simulink model "quad_sim"  (R2016a)
settings: Solver=FixedStepAuto  StartTime=0.0  StopTime=T_sim  FixedStep=dt_sim  RelTol=1e-3
InitFcn:
  | %cd /home/adrianomcr/ROS_projects/vecfield_ws/src/vecfield_lib/simulink/quadrotor
  | MAV_constants
StopFcn:
  | animation
values from neighbouring files (symbols this model uses):
  curva = 9    [MAV_constants.m]
  Delta_omega = 0.5    [MAV_constants.m]
  Delta_tau = 1.0    (= 1)    [MAV_constants.m]
  drag_coef = 0.05    [MAV_constants.m]
  g = 9.81    [MAV_constants.m]
  Kf = 1    [MAV_constants.m]
  Kr = 5    [MAV_constants.m]
  Kv = 2    [MAV_constants.m]
  m = 0.5    [MAV_constants.m]
  Rot_0 = eul2rotm(fliplr([pi/4 pi/2 pi]))    [MAV_constants.m]
  vr = 4    [MAV_constants.m]
  xyz_0 = [-2 -2 -2] + 0.001    [MAV_constants.m]
  xyz_d_0 = [0 1 0] + 0.001    [MAV_constants.m]
settings Model: Creator=root  LastModifiedBy=adrianomcr

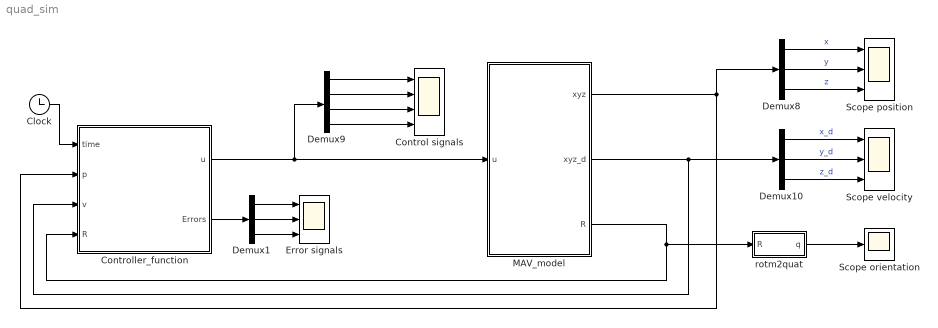
== system quad_sim ==
  Clock : Clock
  Control signals : Scope  NumInputPorts=4
  Controller_function : MATLAB Function  TreatAsAtomicUnit=on
  Demux1 : Demux  Outputs=3
  Demux10 : Demux  Outputs=3
  Demux8 : Demux  Outputs=3
  Demux9 : Demux
  Error signals : Scope  NumInputPorts=3
  MAV_model : Subsystem
  Scope orientation : Scope
  Scope position : Scope  NumInputPorts=3
  Scope velocity : Scope  NumInputPorts=3
  rotm2quat : MATLAB Function  TreatAsAtomicUnit=on
  wires:
  Demux8/1 -> Scope position/1  "x"
  Demux8/2 -> Scope position/2  "y"
  Demux8/3 -> Scope position/3  "z"
  Demux10/1 -> Scope velocity/1  "x_d"
  Demux10/2 -> Scope velocity/2  "y_d"
  Demux10/3 -> Scope velocity/3  "z_d"
  MAV_model/1(xyz) -> Demux8/1, Controller_function/2(p)
  MAV_model/2(xyz_d) -> Controller_function/3(v), Demux10/1
  MAV_model/3(R) -> Controller_function/4(R), rotm2quat/1(R)
  Controller_function/1(u) -> Demux9/1, MAV_model/1(u)
  Demux9/1 -> Control signals/1
  Demux9/2 -> Control signals/2
  Demux9/3 -> Control signals/3
  Demux9/4 -> Control signals/4
  Controller_function/2(Errors) -> Demux1/1
  Demux1/1 -> Error signals/1
  Demux1/2 -> Error signals/2
  Demux1/3 -> Error signals/3
  Clock/1 -> Controller_function/1(time)
  rotm2quat/1(q) -> Scope orientation/1

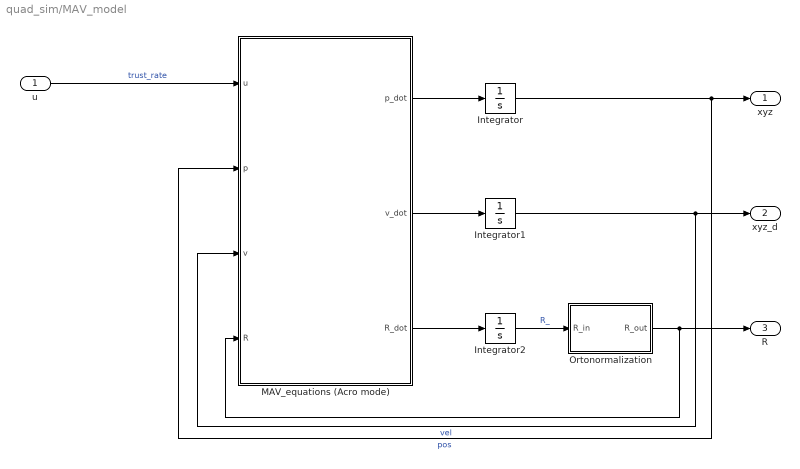
== system quad_sim/MAV_model ==
  u : Inport
  Integrator : Integrator  InitialCondition=xyz_0
  Integrator1 : Integrator  InitialCondition=xyz_d_0
  Integrator2 : Integrator  InitialCondition=Rot_0
  MAV_equations (Acro mode) : MATLAB Function  TreatAsAtomicUnit=on
  Ortonormalization : MATLAB Function  TreatAsAtomicUnit=on
  xyz : Outport
  xyz_d : Outport  Port=2
  R : Outport  Port=3
  wires:
  MAV_equations (Acro mode)/1(p_dot) -> Integrator/1
  MAV_equations (Acro mode)/2(v_dot) -> Integrator1/1
  MAV_equations (Acro mode)/3(R_dot) -> Integrator2/1
  u/1 -> MAV_equations (Acro mode)/1(u)  "trust_rate"
  Integrator2/1 -> Ortonormalization/1(R_in)  "R_"
  Integrator1/1 -> xyz_d/1, MAV_equations (Acro mode)/3(v)  "vel"
  Integrator/1 -> xyz/1, MAV_equations (Acro mode)/2(p)  "pos"
  Ortonormalization/1(R_out) -> R/1, MAV_equations (Acro mode)/4(R)

== matlab function quad_sim/MAV_model/MAV_equations (Acro mode) ==
  data: u input; p_dot output size=3; p input size=3; v input size=3; R input; v_dot output size=3; R_dot output; g parameter; m parameter; drag_coef parameter; Delta_tau parameter; Delta_omega parameter
function [p_dot, v_dot, R_dot] = MAV_equations(u,p,v,R, g, m, drag_coef,Delta_tau, Delta_omega)

%Thrust
tau = u(1);
%Angular velocity
omega = u(2:4); omega = omega(:);

% tau = tau + Delta_tau;
tau = tau + Delta_tau*randn(1);
omega = omega + Delta_omega*randn(3,1);

%Skew-symmetric matrix
S_omega = [   0      -omega(3)  omega(2) ;
           omega(3)      0      -omega(1);
           -omega(2)  omega(1)     0    ];
   
z_hat = [0; 0; 1];

% Drag force
f_drag = -drag_coef*v.*abs(v);


% Model equations
p_dot = v;

v_dot = R*z_hat*tau/m -g*z_hat + f_drag/m;

R_dot = R*S_omega;

== matlab function quad_sim/rotm2quat ==
  data: R input; q output
function q = fcn(R)

q = rotm2quat(R)';

== matlab function quad_sim/MAV_model/Ortonormalization ==
  data: R_in input; R_out output
function R_out = fcn(R_in)

v1 = R_in(:,1);
v2 = R_in(:,2);
v3 = R_in(:,3);

v1 = v1/norm(v1);
v2 = v2 - v1'*v2*v1; v2 = v2/norm(v2);
v3 = cross(v1,v2); v3 = v3/norm(v3);

R_out = [v1,v2,v3];

== matlab function quad_sim/Controller_function ==
  data: time input; p input size=3; v input size=3; R input; u output; vr parameter; m parameter; g parameter; Kv parameter; Kr parameter; Errors output; drag_coef parameter; Kf parameter; curva parameter
function [u, Errors]  = Controller_function(time, p, v, R, vr, m, g, Kv, Kr, drag_coef, Kf, curva)
 

z_b = R(:,3);
z_hat = [0;0;1];

%Vector field
[F, D] = compute_dist_field(p, time, vr, Kf, curva);

psi_r = 0;
% psi_r = atan2(0-p(2),0-p(1));
% psi_r = atan2(F(2),F(1));

%Jacobian of the vector field
[J, Jt] = my_Jacobian(p, time, vr, Kf, curva);

%Drag compensation
f_drag = -drag_coef*v.*abs(v);

%Acceleration reference
a_r = J*v + Kv*(F-v) + Jt + g*z_hat - f_drag/m;

%Computation of reference orientation
z_r = a_r/(norm(a_r)+1e-10);
vec_psi = [cos(psi_r); sin(psi_r); 0];
x_r = (vec_psi - vec_psi'*z_r*z_r)/(norm(vec_psi - vec_psi'*z_r*z_r) + 1e-10);
y_r = cross(z_r,x_r);
Rr = [x_r, y_r, z_r];


%Control law for thrust
tau = m*a_r'*z_b;



%% Recompute values to perform the numeric derivatives
delta_t = 0.05;
p_M = p + v*delta_t;
v_M = v + (z_b*tau/m -g*z_hat + f_drag/m)*delta_t;

[F_M, ~] = compute_dist_field(p_M, time+delta_t, vr, Kf, curva);

psi_r_M = psi_r;
% psi_r_M = atan2(0-p_M(2),0-p_M(1));
% psi_r_M = atan2(F_M(2),F_M(1));

[J_M, Jt_M] = my_Jacobian(p_M, time+delta_t, vr, Kf, curva);

f_drag_M = -drag_coef*v_M.*abs(v_M);

a_r_M = J_M*v_M + Kv*(F_M-v_M) + Jt_M + g*[0;0;1] - f_drag_M/m;

%Computation of reference orientation
z_r_M = a_r_M/(norm(a_r_M)+1e-10);
vec_psi_M = [cos(psi_r_M); sin(psi_r_M); 0];
x_r_M = (vec_psi_M - vec_psi_M'*z_r_M*z_r_M)/(norm(vec_psi_M - vec_psi_M'*z_r_M*z_r_M) + 1e-10);
y_r_M = cross(z_r_M,x_r_M);
Rr_M = [x_r_M, y_r_M, z_r_M];

%% Recompute values to perform the numeric derivatives
p_m = p - v*delta_t;
v_m = v - (z_b*tau/m -g*z_hat + f_drag/m)*delta_t;
% R_M = R;

[F_m, ~] = compute_dist_field(p_m, time-delta_t, vr, Kf, curva);

psi_r_m = psi_r;
% psi_r_m = atan2(0-p_m(2),0-p_m(1));
% psi_r_m = atan2(F_m(2),F_m(1));

[J_m, Jt_m] = my_Jacobian(p_m, time-delta_t, vr, Kf, curva);

f_drag_m = -drag_coef*v_m.*abs(v_m);

a_r_m = J_m*v_m + Kv*(F_m-v_m) + Jt_m + g*[0;0;1] - f_drag_m/m;

%Computation of reference orientation
z_r_m = a_r_m/(norm(a_r_m)+1e-10);
vec_psi_m = [cos(psi_r_m); sin(psi_r_m); 0];
x_r_m = (vec_psi_m - vec_psi_m'*z_r_m*z_r_m)/(norm(vec_psi_m - vec_psi_m'*z_r_m*z_r_m) + 1e-10);
y_r_m = cross(z_r_m,x_r_m);
Rr_m = [x_r_m, y_r_m, z_r_m];



%%

%Orientation error
Re = R'*Rr;

Rr_dot = (Rr_M-Rr_m)/(2*delta_t);
S_w = R'*Rr_dot*Re';
%Feedfoward for omega
omega_d = [S_w(3,2)-S_w(2,3); S_w(1,3)-S_w(3,1); S_w(2,1)-S_w(1,2)]/2;

%Computation of the axis angle representation
n = rotm2axang(Re)';
delta = n(4);
n = n(1:3);

%Control law for the angular rates
omega = omega_d + Kr*sin(delta)*n;

%Ouput errors
Errors = [D, norm(F-v), delta]';

%Output control signals
u = [tau; omega(1); omega(2); omega(3)];
